simulink model "LinearInvertedPendulum"  (R2017a)
settings: Solver=VariableStepAuto  StartTime=0.0  StopTime=10.0  RelTol=1e-3
values from neighbouring files (symbols this model uses):
  g = 9.806    [InvertedPendulum_simulation.m]    (also in linear_CartPend.m; nonlinear_equations.m; solving_equations.m = (m*L^2 + I)/alpha)
  M = 4.800    (= 4.8)    [InvertedPendulum_simulation.m]    (also in nonlinear_equations.m)
  m = 0.356    [InvertedPendulum_simulation.m]    (also in nonlinear_equations.m)
undefined symbols (not defined in the file or in its folder): dmf, fc, l
settings Model: Creator=eddardd  LastModifiedBy=eddardd

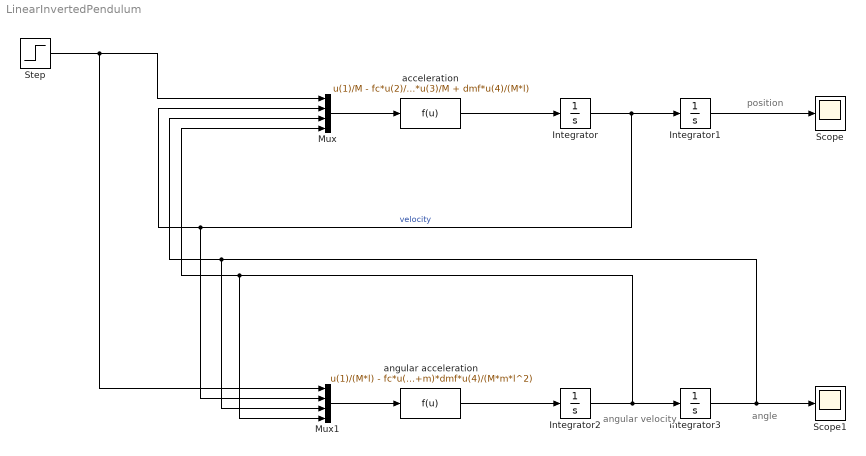
== system LinearInvertedPendulum ==
  note: position
  note: angular velocity
  note: angle
  Integrator{,1..3} (4 alike) : Integrator
  Mux : Mux
  Mux1 : Mux
  Scope : Scope
  Scope1 : Scope
  Step : Step  SampleTime=0
  acceleration : Fcn  Expr=u(1)/M - fc*u(2)/M - m*g*u(3)/M + dmf*u(4)/(M*l)
  angular acceleration : Fcn  Expr=u(1)/(M*l) - fc*u(2)/(M*l) + (M+m)*g*u(3)/(M*l) + (M+m)*dmf*u(4)/(M*m*l^2)
  wires:
  Integrator1/1 -> Scope/1
  Integrator/1 -> Mux1/2, Mux/2, Integrator1/1  "velocity"
  Mux/1 -> acceleration/1
  angular acceleration/1 -> Integrator2/1
  Step/1 -> Mux1/1, Mux/1
  acceleration/1 -> Integrator/1
  Integrator2/1 -> Mux1/4, Mux/4, Integrator3/1
  Mux1/1 -> angular acceleration/1
  Integrator3/1 -> Scope1/1, Mux1/3, Mux/3
